simulink model "E205_Lab4_satellitesim"  (R2014a)
settings: Solver=ode45  StartTime=0.0  StopTime=5  RelTol=1e-3
values from neighbouring files (symbols this model uses):
  J = 2    [E205_Lab4_satellite.m]    (also in satellitescript.m)
  mud = 10    [E205_Lab4_satellite.m]    (also in satellitescript.m)
  mup = 1    [E205_Lab4_satellite.m]    (also in satellitescript.m)
  omegan = 10    [E205_Lab4_satellite.m]    (also in satellitescript.m)
  thetar = r    (= 1)    [E205_Lab4_satellite.m]    (also in satellitescript.m)
  thetardot = 0    [E205_Lab4_satellite.m]    (also in satellitescript.m)
  zeta = 1    [E205_Lab4_satellite.m]    (also in satellitescript.m)
settings Model: Creator=Jessica  LastModifiedBy=Jessica

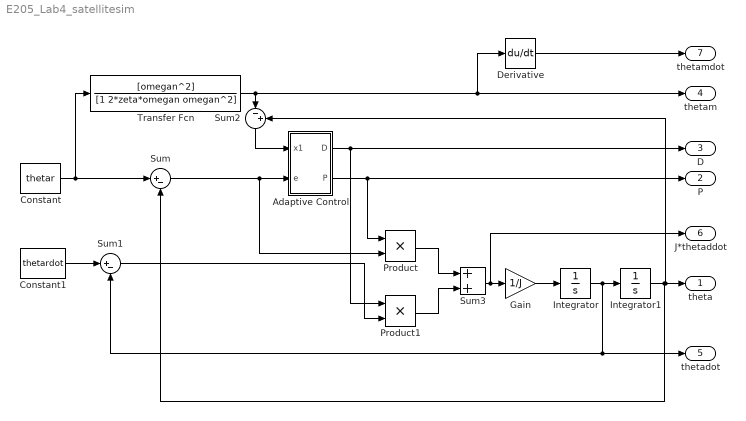
== system E205_Lab4_satellitesim ==
  Adaptive Control : Subsystem
  Constant : Constant  Value=thetar
  Constant1 : Constant  Value=thetardot
  Derivative : Derivative
  Gain : Gain  Gain=1/J
  Integrator : Integrator
  Integrator1 : Integrator
  Product : Product
  Product1 : Product
  Sum : Sum  Inputs=|+-
  Sum1 : Sum  Inputs=|+-
  Sum2 : Sum  Inputs=|-+
  Sum3 : Sum
  Transfer Fcn : TransferFcn  Numerator=[omegan^2]  Denominator=[1 2*zeta*omegan omegan^2]
  theta : Outport
  P : Outport  Port=2
  D : Outport  Port=3
  thetam : Outport  Port=4
  thetadot : Outport  Port=5
  J*thetaddot : Outport  Port=6
  thetamdot : Outport  Port=7
  wires:
  Constant/1 -> Transfer Fcn/1, Sum/1
  Constant1/1 -> Sum1/1
  Transfer Fcn/1 -> Derivative/1, thetam/1, Sum2/1
  Sum2/1 -> Adaptive Control/1(x1)
  Sum/1 -> Product/2, Adaptive Control/2(e)
  Adaptive Control/1(D) -> D/1, Product1/1
  Adaptive Control/2(P) -> P/1, Product/1
  Sum1/1 -> Product1/2
  Product/1 -> Sum3/1
  Product1/1 -> Sum3/2
  Sum3/1 -> J*thetaddot/1, Gain/1
  Gain/1 -> Integrator/1
  Integrator/1 -> thetadot/1, Sum1/2, Integrator1/1
  Integrator1/1 -> Sum2/2, theta/1, Sum/2
  Derivative/1 -> thetamdot/1

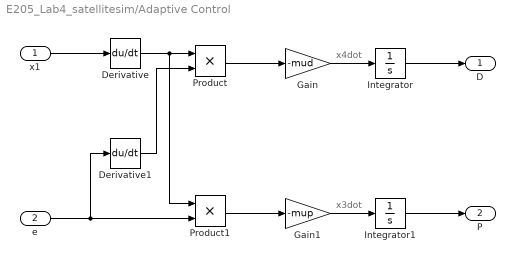
== system E205_Lab4_satellitesim/Adaptive Control ==
  note: x3dot
  note: x4dot
  x1 : Inport
  e : Inport  Port=2
  Derivative : Derivative
  Derivative1 : Derivative
  Gain : Gain  Gain=-mud
  Gain1 : Gain  Gain=-mup
  Integrator : Integrator
  Integrator1 : Integrator
  Product : Product
  Product1 : Product
  D : Outport
  P : Outport  Port=2
  wires:
  Integrator/1 -> D/1
  Product1/1 -> Gain1/1
  Derivative1/1 -> Product/2
  Derivative/1 -> Product1/1, Product/1
  x1/1 -> Derivative/1
  Gain/1 -> Integrator/1
  Gain1/1 -> Integrator1/1
  e/1 -> Product1/2, Derivative1/1
  Integrator1/1 -> P/1
  Product/1 -> Gain/1
